simulink model "Inverse_kinematics_simulink"  (R2022b)
settings: Solver=VariableStepAuto  StartTime=0.0  StopTime=10.0  RelTol=1e-3
settings Model: Creator=Khaled  LastModifiedBy=Khaled

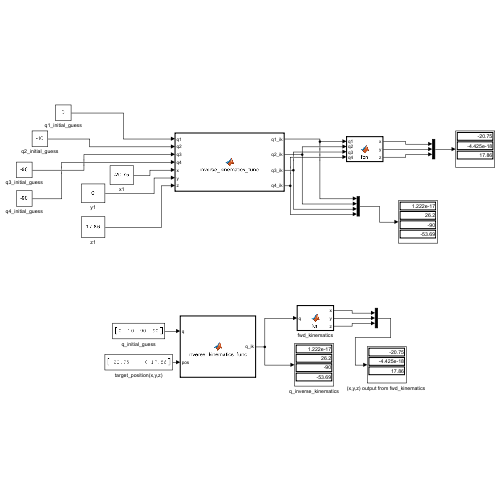
[thumbnail: Simulink's stored preview of the top-level diagram]
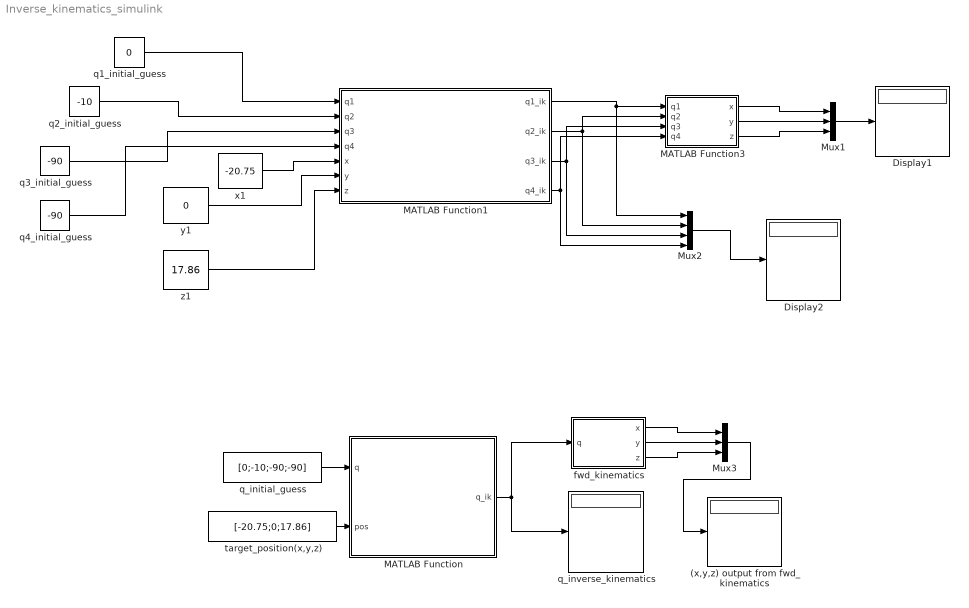
== system Inverse_kinematics_simulink ==
  "(x,y,z) output from fwd_kinematics " : Display
  Display1 : Display
  Display2 : Display
  MATLAB Function : MATLAB Function  TreatAsAtomicUnit=on
  MATLAB Function1 : MATLAB Function  TreatAsAtomicUnit=on
  MATLAB Function3 : MATLAB Function  TreatAsAtomicUnit=on
  Mux1 : Mux  Inputs=3
  Mux2 : Mux
  Mux3 : Mux  Inputs=3
  fwd_kinematics : MATLAB Function  TreatAsAtomicUnit=on
  q1_initial_guess : Constant  Value=0
  q2_initial_guess : Constant  Value=-10
  q3_initial_guess : Constant  Value=-90
  q4_initial_guess : Constant  Value=-90
  q_initial_guess : Constant  Value=[0;-10;-90;-90]
  q_inverse_kinematics : Display
  target_position(x,y,z) : Constant  Value=[-20.75;0;17.86]
  x1 : Constant  Value=-20.75
  y1 : Constant  Value=0
  z1 : Constant  Value=17.86
  wires:
  q_initial_guess/1 -> MATLAB Function/1(q)
  fwd_kinematics/3(z) -> Mux3/3
  MATLAB Function/1(q_ik) -> q_inverse_kinematics/1, fwd_kinematics/1(q)
  Mux3/1 -> "(x,y,z) output from fwd_kinematics "/1
  fwd_kinematics/1(x) -> Mux3/1
  fwd_kinematics/2(y) -> Mux3/2
  MATLAB Function1/2(q2_ik) -> Mux2/2, MATLAB Function3/2(q2)
  q1_initial_guess/1 -> MATLAB Function1/1(q1)
  MATLAB Function1/4(q4_ik) -> MATLAB Function3/4(q4), Mux2/4
  MATLAB Function3/3(z) -> Mux1/3
  q3_initial_guess/1 -> MATLAB Function1/3(q3)
  q2_initial_guess/1 -> MATLAB Function1/2(q2)
  Mux1/1 -> Display1/1
  MATLAB Function3/1(x) -> Mux1/1
  Mux2/1 -> Display2/1
  MATLAB Function1/3(q3_ik) -> MATLAB Function3/3(q3), Mux2/3
  q4_initial_guess/1 -> MATLAB Function1/4(q4)
  MATLAB Function1/1(q1_ik) -> MATLAB Function3/1(q1), Mux2/1
  y1/1 -> MATLAB Function1/6(y)
  z1/1 -> MATLAB Function1/7(z)
  x1/1 -> MATLAB Function1/5(x)
  MATLAB Function3/2(y) -> Mux1/2
  target_position(x,y,z)/1 -> MATLAB Function/2(pos)

== matlab function Inverse_kinematics_simulink/MATLAB Function1 ==
  data: q1 input; q2 input; q3 input; q4 input; q1_ik output; x input; y input; z input; q2_ik output; q3_ik output; q4_ik output
function [q1_ik,q2_ik,q3_ik,q4_ik] = inverse_kinematics_func(q1,q2,q3,q4,x,y,z) 
e = 10^(-2);
pos = [x;y;z];
qo = [q1;q2;q3;q4];
%initially
counter = 0;  
%J_inv_mat = inverse_jacobian_matrix(qo(1),qo(2),qo(3),qo(4));
J1 = [(7*pi*sin((pi*q1)/180)*sin((pi*q2)/180))/90 + (37*pi*cos((pi*q4)/180)*sin((pi*q1)/180)*sin((pi*q2)/180))/450,- (7*pi*cos((pi*q1)/180)*cos((pi*q2)/180))/90 - (37*pi*cos((pi*q1)/180)*cos((pi*q2)/180)*cos((pi*q4)/180))/450, 0, (37*pi*cos((pi*q1)/180)*sin((pi*q2)/180)*sin((pi*q4)/180))/450;
    - (7*pi*cos((pi*q1)/180)*sin((pi*q2)/180))/90 - (37*pi*cos((pi*q1)/180)*cos((pi*q4)/180)*sin((pi*q2)/180))/450, - (7*pi*cos((pi*q2)/180)*sin((pi*q1)/180))/90 - (37*pi*cos((pi*q2)/180)*cos((pi*q4)/180)*sin((pi*q1)/180))/450, 0, (37*pi*sin((pi*q1)/180)*sin((pi*q2)/180)*sin((pi*q4)/180))/450;
    0,                                   - (7*pi*sin((pi*q2)/180))/90 - (37*pi*cos((pi*q4)/180)*sin((pi*q2)/180))/450, 0,                 -(37*pi*cos((pi*q2)/180)*sin((pi*q4)/180))/450];
J2 = [(37*pi*cos((pi*q2)/180)*sin((pi*q1)/180)*sin((pi*q3)/180)*sin((pi*q4)/180))/450 - (37*pi*cos((pi*q1)/180)*cos((pi*q3)/180)*sin((pi*q4)/180))/450, (37*pi*cos((pi*q1)/180)*sin((pi*q2)/180)*sin((pi*q3)/180)*sin((pi*q4)/180))/450,   (37*pi*sin((pi*q1)/180)*sin((pi*q3)/180)*sin((pi*q4)/180))/450 - (37*pi*cos((pi*q1)/180)*cos((pi*q2)/180)*cos((pi*q3)/180)*sin((pi*q4)/180))/450, - (37*pi*cos((pi*q3)/180)*cos((pi*q4)/180)*sin((pi*q1)/180))/450 - (37*pi*cos((pi*q1)/180)*cos((pi*q2)/180)*cos((pi*q4)/180)*sin((pi*q3)/180))/450;
    - (37*pi*cos((pi*q3)/180)*sin((pi*q1)/180)*sin((pi*q4)/180))/450 - (37*pi*cos((pi*q1)/180)*cos((pi*q2)/180)*sin((pi*q3)/180)*sin((pi*q4)/180))/450, (37*pi*sin((pi*q1)/180)*sin((pi*q2)/180)*sin((pi*q3)/180)*sin((pi*q4)/180))/450, - (37*pi*cos((pi*q1)/180)*sin((pi*q3)/180)*sin((pi*q4)/180))/450 - (37*pi*cos((pi*q2)/180)*cos((pi*q3)/180)*sin((pi*q1)/180)*sin((pi*q4)/180))/450,   (37*pi*cos((pi*q1)/180)*cos((pi*q3)/180)*cos((pi*q4)/180))/450 - (37*pi*cos((pi*q2)/180)*cos((pi*q4)/180)*sin((pi*q1)/180)*sin((pi*q3)/180))/450;
    0,                 -(37*pi*cos((pi*q2)/180)*sin((pi*q3)/180)*sin((pi*q4)/180))/450,                                                                                    -(37*pi*cos((pi*q3)/180)*sin((pi*q2)/180)*sin((pi*q4)/180))/450,                                                                                    -(37*pi*cos((pi*q4)/180)*sin((pi*q2)/180)*sin((pi*q3)/180))/450];

J_f = J1+J2;
J_inv_mat = pinv(J_f);
fwd_mat_value = forward_kinematics_func_num(qo(1),qo(2),qo(3),qo(4));
fwd_mat_value = fwd_mat_value - pos;
q_new = qo - (J_inv_mat*fwd_mat_value);
error = abs(fwd_mat_value);

  while(error(1)>=e || error(2)>=e || error(3)>=e)
      q_n = q_new;
      %J_inv_mat = inverse_jacobian_matrix(q_n(1),q_n(2),q_n(3),q_n(4));
      J1 = [(7*pi*sin((pi*q1)/180)*sin((pi*q2)/180))/90 + (37*pi*cos((pi*q4)/180)*sin((pi*q1)/180)*sin((pi*q2)/180))/450,- (7*pi*cos((pi*q1)/180)*cos((pi*q2)/180))/90 - (37*pi*cos((pi*q1)/180)*cos((pi*q2)/180)*cos((pi*q4)/180))/450, 0, (37*pi*cos((pi*q1)/180)*sin((pi*q2)/180)*sin((pi*q4)/180))/450;
    - (7*pi*cos((pi*q1)/180)*sin((pi*q2)/180))/90 - (37*pi*cos((pi*q1)/180)*cos((pi*q4)/180)*sin((pi*q2)/180))/450, - (7*pi*cos((pi*q2)/180)*sin((pi*q1)/180))/90 - (37*pi*cos((pi*q2)/180)*cos((pi*q4)/180)*sin((pi*q1)/180))/450, 0, (37*pi*sin((pi*q1)/180)*sin((pi*q2)/180)*sin((pi*q4)/180))/450;
    0,                                   - (7*pi*sin((pi*q2)/180))/90 - (37*pi*cos((pi*q4)/180)*sin((pi*q2)/180))/450, 0,                 -(37*pi*cos((pi*q2)/180)*sin((pi*q4)/180))/450];
J2 = [(37*pi*cos((pi*q2)/180)*sin((pi*q1)/180)*sin((pi*q3)/180)*sin((pi*q4)/180))/450 - (37*pi*cos((pi*q1)/180)*cos((pi*q3)/180)*sin((pi*q4)/180))/450, (37*pi*cos((pi*q1)/180)*sin((pi*q2)/180)*sin((pi*q3)/180)*sin((pi*q4)/180))/450,   (37*pi*sin((pi*q1)/180)*sin((pi*q3)/180)*sin((pi*q4)/180))/450 - (37*pi*cos((pi*q1)/180)*cos((pi*q2)/180)*cos((pi*q3)/180)*sin((pi*q4)/180))/450, - (37*pi*cos((pi*q3)/180)*cos((pi*q4)/180)*sin((pi*q1)/180))/450 - (37*pi*cos((pi*q1)/180)*cos((pi*q2)/180)*cos((pi*q4)/180)*sin((pi*q3)/180))/450;
    - (37*pi*cos((pi*q3)/180)*sin((pi*q1)/180)*sin((pi*q4)/180))/450 - (37*pi*cos((pi*q1)/180)*cos((pi*q2)/180)*sin((pi*q3)/180)*sin((pi*q4)/180))/450, (37*pi*sin((pi*q1)/180)*sin((pi*q2)/180)*sin((pi*q3)/180)*sin((pi*q4)/180))/450, - (37*pi*cos((pi*q1)/180)*sin((pi*q3)/180)*sin((pi*q4)/180))/450 - (37*pi*cos((pi*q2)/180)*cos((pi*q3)/180)*sin((pi*q1)/180)*sin((pi*q4)/180))/450,   (37*pi*cos((pi*q1)/180)*cos((pi*q3)/180)*cos((pi*q4)/180))/450 - (37*pi*cos((pi*q2)/180)*cos((pi*q4)/180)*sin((pi*q1)/180)*sin((pi*q3)/180))/450;
    0,                 -(37*pi*cos((pi*q2)/180)*sin((pi*q3)/180)*sin((pi*q4)/180))/450,                                                                                    -(37*pi*cos((pi*q3)/180)*sin((pi*q2)/180)*sin((pi*q4)/180))/450,                                                                                    -(37*pi*cos((pi*q4)/180)*sin((pi*q2)/180)*sin((pi*q3)/180))/450];

J_f = J1+J2;
J_inv_mat = pinv(J_f);
      fwd_mat_value = forward_kinematics_func_num(q_n(1),q_n(2),q_n(3),q_n(4));
      fwd_mat_value = fwd_mat_value - pos;
      q_new = q_n - J_inv_mat*fwd_mat_value;
      error = abs(fwd_mat_value);
      counter=counter+1;
  end
  q1_ik = q_new(1);
  q2_ik = q_new(2);
  q3_ik = q_new(3);
  q4_ik = q_new(4);
end

== matlab function Inverse_kinematics_simulink/MATLAB Function ==
  data: q input; q_ik output; pos input
function q_ik = inverse_kinematics_func(q,pos) 
q1 = q(1);
q2 = q(2);
q3 = q(3);
q4 = q(4);
e = 10^(-2);
%pos = [x;y;z];
qo = [q1;q2;q3;q4];
%initially
counter = 0;  
%J_inv_mat = inverse_jacobian_matrix(qo(1),qo(2),qo(3),qo(4));
J1 = [(7*pi*sin((pi*q1)/180)*sin((pi*q2)/180))/90 + (37*pi*cos((pi*q4)/180)*sin((pi*q1)/180)*sin((pi*q2)/180))/450,- (7*pi*cos((pi*q1)/180)*cos((pi*q2)/180))/90 - (37*pi*cos((pi*q1)/180)*cos((pi*q2)/180)*cos((pi*q4)/180))/450, 0, (37*pi*cos((pi*q1)/180)*sin((pi*q2)/180)*sin((pi*q4)/180))/450;
    - (7*pi*cos((pi*q1)/180)*sin((pi*q2)/180))/90 - (37*pi*cos((pi*q1)/180)*cos((pi*q4)/180)*sin((pi*q2)/180))/450, - (7*pi*cos((pi*q2)/180)*sin((pi*q1)/180))/90 - (37*pi*cos((pi*q2)/180)*cos((pi*q4)/180)*sin((pi*q1)/180))/450, 0, (37*pi*sin((pi*q1)/180)*sin((pi*q2)/180)*sin((pi*q4)/180))/450;
    0,                                   - (7*pi*sin((pi*q2)/180))/90 - (37*pi*cos((pi*q4)/180)*sin((pi*q2)/180))/450, 0,                 -(37*pi*cos((pi*q2)/180)*sin((pi*q4)/180))/450];
J2 = [(37*pi*cos((pi*q2)/180)*sin((pi*q1)/180)*sin((pi*q3)/180)*sin((pi*q4)/180))/450 - (37*pi*cos((pi*q1)/180)*cos((pi*q3)/180)*sin((pi*q4)/180))/450, (37*pi*cos((pi*q1)/180)*sin((pi*q2)/180)*sin((pi*q3)/180)*sin((pi*q4)/180))/450,   (37*pi*sin((pi*q1)/180)*sin((pi*q3)/180)*sin((pi*q4)/180))/450 - (37*pi*cos((pi*q1)/180)*cos((pi*q2)/180)*cos((pi*q3)/180)*sin((pi*q4)/180))/450, - (37*pi*cos((pi*q3)/180)*cos((pi*q4)/180)*sin((pi*q1)/180))/450 - (37*pi*cos((pi*q1)/180)*cos((pi*q2)/180)*cos((pi*q4)/180)*sin((pi*q3)/180))/450;
    - (37*pi*cos((pi*q3)/180)*sin((pi*q1)/180)*sin((pi*q4)/180))/450 - (37*pi*cos((pi*q1)/180)*cos((pi*q2)/180)*sin((pi*q3)/180)*sin((pi*q4)/180))/450, (37*pi*sin((pi*q1)/180)*sin((pi*q2)/180)*sin((pi*q3)/180)*sin((pi*q4)/180))/450, - (37*pi*cos((pi*q1)/180)*sin((pi*q3)/180)*sin((pi*q4)/180))/450 - (37*pi*cos((pi*q2)/180)*cos((pi*q3)/180)*sin((pi*q1)/180)*sin((pi*q4)/180))/450,   (37*pi*cos((pi*q1)/180)*cos((pi*q3)/180)*cos((pi*q4)/180))/450 - (37*pi*cos((pi*q2)/180)*cos((pi*q4)/180)*sin((pi*q1)/180)*sin((pi*q3)/180))/450;
    0,                 -(37*pi*cos((pi*q2)/180)*sin((pi*q3)/180)*sin((pi*q4)/180))/450,                                                                                    -(37*pi*cos((pi*q3)/180)*sin((pi*q2)/180)*sin((pi*q4)/180))/450,                                                                                    -(37*pi*cos((pi*q4)/180)*sin((pi*q2)/180)*sin((pi*q3)/180))/450];

J_f = J1+J2;
J_inv_mat = pinv(J_f);
fwd_mat_value = forward_kinematics_func_num(qo(1),qo(2),qo(3),qo(4));
fwd_mat_value = fwd_mat_value - pos;
q_new = qo - (J_inv_mat*fwd_mat_value);
error = abs(fwd_mat_value);

  while(error(1)>=e || error(2)>=e || error(3)>=e)
      q_n = q_new;
      %J_inv_mat = inverse_jacobian_matrix(q_n(1),q_n(2),q_n(3),q_n(4));
      J1 = [(7*pi*sin((pi*q1)/180)*sin((pi*q2)/180))/90 + (37*pi*cos((pi*q4)/180)*sin((pi*q1)/180)*sin((pi*q2)/180))/450,- (7*pi*cos((pi*q1)/180)*cos((pi*q2)/180))/90 - (37*pi*cos((pi*q1)/180)*cos((pi*q2)/180)*cos((pi*q4)/180))/450, 0, (37*pi*cos((pi*q1)/180)*sin((pi*q2)/180)*sin((pi*q4)/180))/450;
    - (7*pi*cos((pi*q1)/180)*sin((pi*q2)/180))/90 - (37*pi*cos((pi*q1)/180)*cos((pi*q4)/180)*sin((pi*q2)/180))/450, - (7*pi*cos((pi*q2)/180)*sin((pi*q1)/180))/90 - (37*pi*cos((pi*q2)/180)*cos((pi*q4)/180)*sin((pi*q1)/180))/450, 0, (37*pi*sin((pi*q1)/180)*sin((pi*q2)/180)*sin((pi*q4)/180))/450;
    0,                                   - (7*pi*sin((pi*q2)/180))/90 - (37*pi*cos((pi*q4)/180)*sin((pi*q2)/180))/450, 0,                 -(37*pi*cos((pi*q2)/180)*sin((pi*q4)/180))/450];
J2 = [(37*pi*cos((pi*q2)/180)*sin((pi*q1)/180)*sin((pi*q3)/180)*sin((pi*q4)/180))/450 - (37*pi*cos((pi*q1)/180)*cos((pi*q3)/180)*sin((pi*q4)/180))/450, (37*pi*cos((pi*q1)/180)*sin((pi*q2)/180)*sin((pi*q3)/180)*sin((pi*q4)/180))/450,   (37*pi*sin((pi*q1)/180)*sin((pi*q3)/180)*sin((pi*q4)/180))/450 - (37*pi*cos((pi*q1)/180)*cos((pi*q2)/180)*cos((pi*q3)/180)*sin((pi*q4)/180))/450, - (37*pi*cos((pi*q3)/180)*cos((pi*q4)/180)*sin((pi*q1)/180))/450 - (37*pi*cos((pi*q1)/180)*cos((pi*q2)/180)*cos((pi*q4)/180)*sin((pi*q3)/180))/450;
    - (37*pi*cos((pi*q3)/180)*sin((pi*q1)/180)*sin((pi*q4)/180))/450 - (37*pi*cos((pi*q1)/180)*cos((pi*q2)/180)*sin((pi*q3)/180)*sin((pi*q4)/180))/450, (37*pi*sin((pi*q1)/180)*sin((pi*q2)/180)*sin((pi*q3)/180)*sin((pi*q4)/180))/450, - (37*pi*cos((pi*q1)/180)*sin((pi*q3)/180)*sin((pi*q4)/180))/450 - (37*pi*cos((pi*q2)/180)*cos((pi*q3)/180)*sin((pi*q1)/180)*sin((pi*q4)/180))/450,   (37*pi*cos((pi*q1)/180)*cos((pi*q3)/180)*cos((pi*q4)/180))/450 - (37*pi*cos((pi*q2)/180)*cos((pi*q4)/180)*sin((pi*q1)/180)*sin((pi*q3)/180))/450;
    0,                 -(37*pi*cos((pi*q2)/180)*sin((pi*q3)/180)*sin((pi*q4)/180))/450,                                                                                    -(37*pi*cos((pi*q3)/180)*sin((pi*q2)/180)*sin((pi*q4)/180))/450,                                                                                    -(37*pi*cos((pi*q4)/180)*sin((pi*q2)/180)*sin((pi*q3)/180))/450];

J_f = J1+J2;
J_inv_mat = pinv(J_f);
      fwd_mat_value = forward_kinematics_func_num(q_n(1),q_n(2),q_n(3),q_n(4));
      fwd_mat_value = fwd_mat_value - pos;
      q_new = q_n - J_inv_mat*fwd_mat_value;
      error = abs(fwd_mat_value);
      counter=counter+1;
  end
  q_ik = q_new;
end

== matlab function Inverse_kinematics_simulink/fwd_kinematics ==
  data: q input; x output; y output; z output
function [x,y,z] = fcn(q)
q1 = q(1);
q2 = q(2);
q3 = q(3);
q4 = q(4);
T1 = Transformation_func(q1,2.7,0,90);
T2 = Transformation_func(q2,0,0,-90);
T3 = Transformation_func(q3+90,14,0,-90);
T4 = Transformation_func(q4-90,0,14.8,0);
TT = T1*T2*T3*T4;
x = TT(1,4);
y = TT(2,4);
z = TT(3,4);
end

== matlab function Inverse_kinematics_simulink/MATLAB Function3 ==
  data: q1 input; x output; y output; z output; q2 input; q3 input; q4 input
function [x,y,z] = fcn(q1,q2,q3,q4)
T1 = Transformation_func(q1,2.7,0,90);
T2 = Transformation_func(q2,0,0,-90);
T3 = Transformation_func(q3+90,14,0,-90);
T4 = Transformation_func(q4-90,0,14.8,0);
TT = T1*T2*T3*T4;
x = TT(1,4);
y = TT(2,4);
z = TT(3,4);
end
